simulink model "Question12_22104137"  (R2022a)
settings: Solver=ode3  StartTime=0.0  StopTime=0.5  FixedStep=T  RelTol=1e-3
InitFcn:
  | T=5e-6
  | fsw=1550
  | Ts=1/fsw
libraries: spsDiodeLib x18, spsIGBTDiodeLib x8, spsCurrentMeasurementLib x7, spsSeriesRLCBranchLib x7, simulink x6, spsVoltageMeasurementLib x4, spsMeanLib x3, spsMultiWindingTransformerLib x3, spsThreePhaseSourceLib x1, spspowerguiLib x1
settings Model: Creator=vinay  LastModifiedBy=vinay
settings DataIOCC: SaveFormat=StructureWithTime  ReturnWorkspaceOutputs=off
settings ModelReferenceCC: EnableRefExpFcnMdlSchedulingChecks=off
settings RTWCC: Description=Generic Real-Time Target

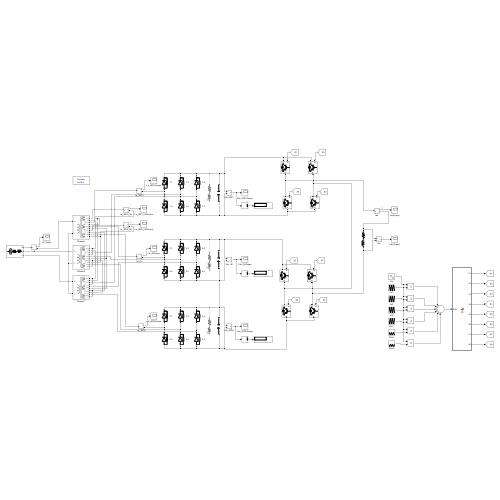
[thumbnail: Simulink's stored preview of the top-level diagram]
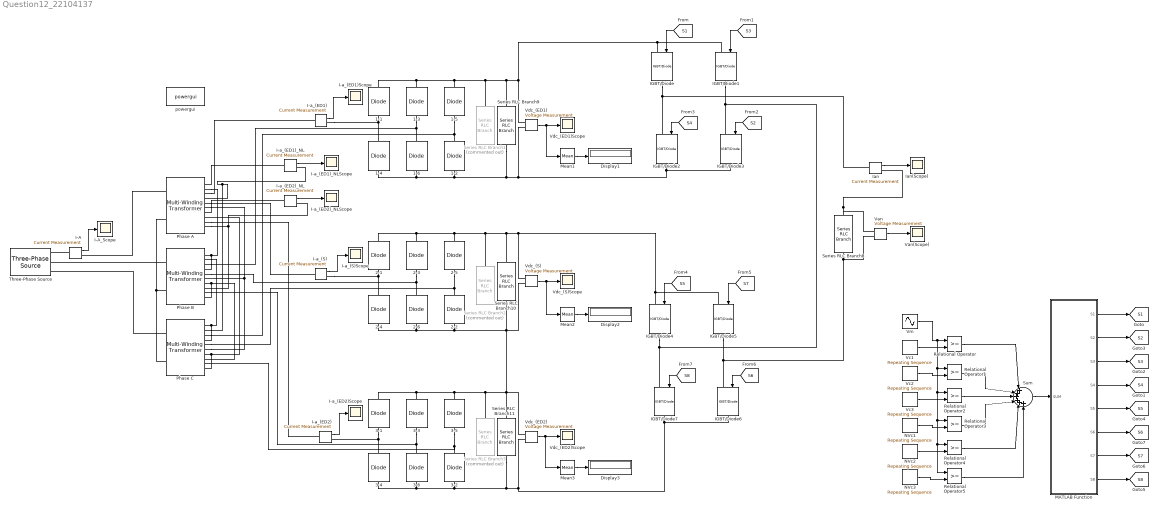
== system Question12_22104137 ==
  1-{1..6} (6 alike) : spsDiodeLib/Diode  Ron=0.001  Lon=0  Vf=0.8  IC=0  UseSnubber=0  Rs=500  Cs=250e-9  Measurements=off
  2-{1..6} (6 alike) : spsDiodeLib/Diode  Ron=0.001  Lon=0  Vf=0.8  IC=0  UseSnubber=0  Rs=500  Cs=250e-9  Measurements=off
  3-{1..6} (6 alike) : spsDiodeLib/Diode  Ron=0.001  Lon=0  Vf=0.8  IC=0  UseSnubber=0  Rs=500  Cs=250e-9  Measurements=off
  Display1 : Display
  Display2 : Display
  Display3 : Display
  I-A : spsCurrentMeasurementLib/Current Measurement  PhasorSimulation=off  OutputType=Complex  PSBequivalent=0
  I-A_Scope : Scope
  I-a_(ED1) : spsCurrentMeasurementLib/Current Measurement  PhasorSimulation=off  OutputType=Complex  PSBequivalent=0
  I-a_(ED1)Scope : Scope
  I-a_(ED1)_NL : spsCurrentMeasurementLib/Current Measurement  PhasorSimulation=off  OutputType=Complex  PSBequivalent=0
  I-a_(ED1)_NLScope : Scope
  I-a_(ED2) : spsCurrentMeasurementLib/Current Measurement  PhasorSimulation=off  OutputType=Complex  PSBequivalent=0
  I-a_(ED2)Scope : Scope
  I-a_(ED2)_NL : spsCurrentMeasurementLib/Current Measurement  PhasorSimulation=off  OutputType=Complex  PSBequivalent=0
  I-a_(ED2)_NLScope : Scope
  I-a_(S) : spsCurrentMeasurementLib/Current Measurement  PhasorSimulation=off  OutputType=Complex  PSBequivalent=0
  I-a_(S)Scope : Scope
  IGBT/Diode{,1..7} (8 alike) : spsIGBTDiodeLib/IGBT//Diode  Ron=1e-3  Rs=1e5  Cs=inf  Measurements=off
  Ian : spsCurrentMeasurementLib/Current Measurement  PhasorSimulation=off  OutputType=Complex  PSBequivalent=0
  Ian(Scope) : Scope
  MATLAB Function : MATLAB Function  TreatAsAtomicUnit=on
  Mean1 : spsMeanLib/Mean  Freq=50  Vinit=0  Ts=0
  Mean2 : spsMeanLib/Mean  Freq=50  Vinit=0  Ts=0
  Mean3 : spsMeanLib/Mean  Freq=50  Vinit=0  Ts=0
  NVc1 : simulink/Sources/Repeating Sequence  rep_seq_t=[0 1/2 1]*Ts  rep_seq_y=[0 -1 0]
  NVc2 : simulink/Sources/Repeating Sequence  rep_seq_t=[0 1/2 1]*Ts  rep_seq_y=[-2 -1 -2]
  NVc3 : simulink/Sources/Repeating Sequence  rep_seq_t=[0 1/2 1]*Ts  rep_seq_y=[-2 -3 -2]
  Phase A : spsMultiWindingTransformerLib/Multi-Winding Transformer  LeftWindings=1  RightWindings=5  TappedWindings=no taps  NumberOfTaps=2  SetSaturation=off  Hysteresis=off  DataFile='hysteresis.mat'  Measurements=None  UNITS=pu  NominalPower=[2.5e3 50]  NominalVoltages="[ 239.6  78.8  45.5  86  78.8  45.5 ]"  WindingResistances="[ 0  0  0  0  0  0 ]"  WindingInductances="[ 0.09  0.09  0.09  0.09  0.09  0.09 ]"  Rm=500  Lm=500  Saturation=[ 0,0 ; 0.0024,1.2 ; 1.0,1.52 ]  SpecifyInitialFlux=off  InitialFlux=0  BreakLoop=off  DiscreteSolver=Trapezoidal iterative  DataType=off  TransfoNumber=1
  Phase B : spsMultiWindingTransformerLib/Multi-Winding Transformer  LeftWindings=1  RightWindings=5  TappedWindings=no taps  NumberOfTaps=2  SetSaturation=off  Hysteresis=off  DataFile='hysteresis.mat'  Measurements=None  UNITS=pu  NominalPower=[2.5e3 50]  NominalVoltages="[ 239.6  78.8  45.5  86  78.8  45.5 ]"  WindingResistances="[ 0  0  0  0  0  0 ]"  WindingInductances="[ 0.09  0.09  0.09  0.09  0.09  0.09 ]"  Rm=500  Lm=500  Saturation=[ 0,0 ; 0.0024,1.2 ; 1.0,1.52 ]  SpecifyInitialFlux=off  InitialFlux=0  BreakLoop=off  DiscreteSolver=Trapezoidal iterative  DataType=off  TransfoNumber=1
  Phase C : spsMultiWindingTransformerLib/Multi-Winding Transformer  LeftWindings=1  RightWindings=5  TappedWindings=no taps  NumberOfTaps=2  SetSaturation=off  Hysteresis=off  DataFile='hysteresis.mat'  Measurements=None  UNITS=pu  NominalPower=[2.5e3 50]  NominalVoltages="[ 239.6  78.8  45.5  86  78.8  45.5 ]"  WindingResistances="[ 0  0  0  0  0  0 ]"  WindingInductances="[ 0.09  0.09  0.09  0.09  0.09  0.09 ]"  Rm=500  Lm=500  Saturation=[ 0,0 ; 0.0024,1.2 ; 1.0,1.52 ]  SpecifyInitialFlux=off  InitialFlux=0  BreakLoop=off  DiscreteSolver=Trapezoidal iterative  DataType=off  TransfoNumber=1
  Relational Operator{,1..5} (6 alike) : RelationalOperator  OutDataTypeStr=boolean  RndMeth=Simplest  InputSameDT=off
  Series RLC Branch1 : spsSeriesRLCBranchLib/Series RLC Branch  Commented=on  LConnTagsString=__new0  RConnTagsString=__new0  BranchType=RL  Resistance=50  Inductance=100e-3  SetiL0=off  InitialCurrent=0  Capacitance=1e-6  Setx0=off  InitialVoltage=0  Measurements=None
  Series RLC Branch10 : spsSeriesRLCBranchLib/Series RLC Branch  LConnTagsString=__new0  RConnTagsString=__new0  BranchType=C  Resistance=1  Inductance=1e-3  SetiL0=off  InitialCurrent=0  Capacitance=4700e-6  Setx0=off  InitialVoltage=0  Measurements=None
  Series RLC Branch11 : spsSeriesRLCBranchLib/Series RLC Branch  LConnTagsString=__new0  RConnTagsString=__new0  BranchType=C  Resistance=1  Inductance=1e-3  SetiL0=off  InitialCurrent=0  Capacitance=4700e-6  Setx0=off  InitialVoltage=0  Measurements=None
  Series RLC Branch2 : spsSeriesRLCBranchLib/Series RLC Branch  Commented=on  LConnTagsString=__new0  RConnTagsString=__new0  BranchType=RL  Resistance=50  Inductance=100e-3  SetiL0=off  InitialCurrent=0  Capacitance=1e-6  Setx0=off  InitialVoltage=0  Measurements=None
  Series RLC Branch3 : spsSeriesRLCBranchLib/Series RLC Branch  Commented=on  LConnTagsString=__new0  RConnTagsString=__new0  BranchType=RL  Resistance=50  Inductance=100e-3  SetiL0=off  InitialCurrent=0  Capacitance=1e-6  Setx0=off  InitialVoltage=0  Measurements=None
  Series RLC Branch8 : spsSeriesRLCBranchLib/Series RLC Branch  LConnTagsString=__new0  RConnTagsString=__new0  BranchType=RL  Resistance=50  Inductance=10e-3  SetiL0=off  InitialCurrent=0  Capacitance=1e-6  Setx0=off  InitialVoltage=0  Measurements=None
  Series RLC Branch9 : spsSeriesRLCBranchLib/Series RLC Branch  LConnTagsString=__new0  RConnTagsString=__new0  BranchType=C  Resistance=1  Inductance=1e-3  SetiL0=off  InitialCurrent=0  Capacitance=4700e-6  Setx0=off  InitialVoltage=0  Measurements=None
  Sum : Sum  Inputs=|++++++
  Three-Phase Source : spsThreePhaseSourceLib/Three-Phase Source  InternalConnection=Y  VoltagePhases=on  Voltage=415  PhaseAngle=0  Voltage_phases=[415 415 415]/sqrt(3)  PhaseAngles_phases=[0 120 240]  Frequency=50  NonIdealSource=on  SpecifyImpedance=off  Resistance=0.001  Inductance=5e-6  ShortCircuitLevel=100e6  BaseVoltage=415  XRratio=7  BusType=swing  Pref=10e3  Qref=0  Prefabc=[10e3, 10e3, 10e3]  Qrefabc=[0, 0, 0]  Qmin=-inf  Qmax=inf
  Van : spsVoltageMeasurementLib/Voltage Measurement  PhasorSimulation=off  OutputType=Complex  PSBequivalent=0
  Van(Scope) : Scope
  Vc1 : simulink/Sources/Repeating Sequence  rep_seq_t=[0 1/2 1]*Ts  rep_seq_y=[0 1 0]
  Vc2 : simulink/Sources/Repeating Sequence  rep_seq_t=[0 1/2 1]*Ts  rep_seq_y=[2 1 2]
  Vc3 : simulink/Sources/Repeating Sequence  rep_seq_t=[0 1/2 1]*Ts  rep_seq_y=[2 3 2]
  Vdc_(ED1) : spsVoltageMeasurementLib/Voltage Measurement  PhasorSimulation=off  OutputType=Complex  PSBequivalent=0
  Vdc_(ED1)Scope : Scope
  Vdc_(ED2) : spsVoltageMeasurementLib/Voltage Measurement  PhasorSimulation=off  OutputType=Complex  PSBequivalent=0
  Vdc_(ED2)Scope : Scope
  Vdc_(S) : spsVoltageMeasurementLib/Voltage Measurement  PhasorSimulation=off  OutputType=Complex  PSBequivalent=0
  Vdc_(S)Scope : Scope
  Vm : Sin  Amplitude=3  Frequency=2*pi*50  SampleTime=0
  powergui : spspowerguiLib/powergui  Priority=1  SimulationMode=Discrete  SampleTime=T  frequency=60  Iterations=50  frequencyindice=0  Pbase=100e6  ErrMax=1e-4  UnitsV=kV  UnitsW=MW  buscounter=0  FunctionMessages=off  echomessages=off  EnableUseOfTLC=off  CurrentSourceSwitches=off  DisableSnubberDevices=off  DisableRonSwitches=off  DisableVfSwitches=off  DisplayEquations=off  AutomaticDiscreteSolvers=off  SolverType=Tustin/Backward Euler (TBE)  Interpol=off  ExternalGateDelay=off  methode=off  Ts=100  x0status=blocks  SPID=on  SwTol=0  HookPort=off  NonlinearTolerance=1e-4  nMaxIteration=100  ContinueOnMaxIteration=off  RestoreLinks=warning  ResistiveCurrentMeasurement=off  Frange=[0:2:500]  Ylog=off  Xlog=on  ShowGrid=off  save=off  variable=ZData  structure=0  ZoomFFT=off  StartTime=0.0  cycles=1  DisplayStyle=1  fundamental=60  FreqAxis=off  MaxFrequency=1000  frequencyindicesteady=1  RmsSteady=1  display=off
  tag scope: S1=global, S2=global, S3=global, S4=global, S5=global, S6=global, S7=global, S8=global
  wires:
  Vdc_(ED1)/1 -> Vdc_(ED1)Scope/1, Mean1/1
  Mean1/1 -> Display1/1
  Vdc_(S)/1 -> Vdc_(S)Scope/1, Mean2/1
  Mean2/1 -> Display2/1
  Vdc_(ED2)/1 -> Vdc_(ED2)Scope/1, Mean3/1
  Mean3/1 -> Display3/1
  I-a_(ED1)/1 -> I-a_(ED1)Scope/1
  I-a_(S)/1 -> I-a_(S)Scope/1
  I-a_(ED2)/1 -> I-a_(ED2)Scope/1
  Van/1 -> Van(Scope)/1
  [S6] -> IGBT/Diode6/1
  [S7] -> IGBT/Diode5/1
  [S5] -> IGBT/Diode4/1
  Ian/1 -> Ian(Scope)/1
  [S2] -> IGBT/Diode3/1
  [S4] -> IGBT/Diode2/1
  [S8] -> IGBT/Diode7/1
  [S3] -> IGBT/Diode1/1
  [S1] -> IGBT/Diode/1
  I-A/1 -> I-A_Scope/1
  Vm/1 -> Relational Operator5/1, Relational Operator4/1, Relational Operator3/1, Relational Operator2/1, Relational Operator1/1, Relational Operator/1
  NVc3/1 -> Relational Operator5/2
  NVc2/1 -> Relational Operator4/2
  NVc1/1 -> Relational Operator3/2
  Vc3/1 -> Relational Operator2/2
  Vc2/1 -> Relational Operator1/2
  Vc1/1 -> Relational Operator/2
  Relational Operator/1 -> Sum/1
  Relational Operator1/1 -> Sum/2
  Relational Operator2/1 -> Sum/3
  Relational Operator3/1 -> Sum/4
  Relational Operator4/1 -> Sum/5
  Relational Operator5/1 -> Sum/6
  Sum/1 -> MATLAB Function/1(SUM)
  MATLAB Function/6(S6) -> [S6]
  MATLAB Function/1(S1) -> [S1]
  MATLAB Function/2(S2) -> [S2]
  MATLAB Function/3(S3) -> [S3]
  MATLAB Function/4(S4) -> [S4]
  MATLAB Function/5(S5) -> [S5]
  MATLAB Function/7(S7) -> [S7]
  MATLAB Function/8(S8) -> [S8]
  I-a_(ED1)_NL/1 -> I-a_(ED1)_NLScope/1
  I-a_(ED2)_NL/1 -> I-a_(ED2)_NLScope/1
  connections:
  1-1/LConn1 -- 1-4/RConn1 -- I-a_(ED1)/RConn1
  1-5/LConn1 -- Phase C/RConn3 -- 1-2/RConn1
  1-3/LConn1 -- Phase B/RConn3 -- 1-6/RConn1
  3-1/LConn1 -- 3-4/RConn1 -- I-a_(ED2)/RConn1
  3-5/LConn1 -- Phase C/RConn9 -- 3-2/RConn1
  3-3/LConn1 -- Phase B/RConn9 -- 3-6/RConn1
  2-1/LConn1 -- 2-4/RConn1 -- I-a_(S)/RConn1
  2-3/LConn1 -- Phase B/RConn5 -- 2-6/RConn1
  2-5/LConn1 -- Phase C/RConn5 -- 2-2/RConn1
  Vdc_(ED2)/LConn1 -- Series RLC Branch11/LConn1 -- Series RLC Branch10/RConn1 -- Vdc_(S)/LConn2 -- 2-4/LConn1 -- 2-6/LConn1 -- 2-2/LConn1 -- Series RLC Branch3/LConn1 -- 3-3/RConn1 -- 3-1/RConn1 -- 3-5/RConn1
  Ian/LConn1 -- IGBT/Diode2/LConn1 -- IGBT/Diode/RConn1
  Series RLC Branch8/RConn1 -- IGBT/Diode6/LConn1 -- IGBT/Diode5/RConn1 -- Van/LConn2
  IGBT/Diode7/LConn1 -- IGBT/Diode4/RConn1 -- IGBT/Diode3/LConn1 -- IGBT/Diode1/RConn1
  Phase B/LConn2 -- Phase A/LConn2 -- Phase C/LConn2
  Phase C/LConn1 -- Three-Phase Source/RConn3
  Phase A/LConn1 -- I-A/RConn1
  Phase B/LConn1 -- Three-Phase Source/RConn2
  I-A/LConn1 -- Three-Phase Source/RConn1
  Phase A/RConn1 -- I-a_(ED1)_NL/LConn1
  Phase B/RConn1 -- Phase A/RConn2 -- Phase B/RConn4
  Phase C/RConn1 -- Phase B/RConn2 -- Phase C/RConn4
  Phase A/RConn10 -- I-a_(ED2)_NL/RConn1 -- Phase B/RConn8
  Phase B/RConn7 -- Phase B/RConn10 -- Phase C/RConn8
  Phase C/RConn7 -- Phase C/RConn10 -- Phase A/RConn8
  Phase A/RConn6 -- Phase C/RConn6 -- Phase B/RConn6
  Phase A/RConn3 -- I-a_(ED1)/LConn1
  Phase A/RConn5 -- I-a_(S)/LConn1
  Phase A/RConn9 -- I-a_(ED2)/LConn1
  IGBT/Diode6/RConn1 -- Series RLC Branch11/RConn1 -- 3-2/LConn1 -- 3-4/LConn1 -- 3-6/LConn1 -- Vdc_(ED2)/LConn2 -- IGBT/Diode7/RConn1
  2-5/RConn1 -- Series RLC Branch2/LConn1 -- Vdc_(S)/LConn1 -- IGBT/Diode5/LConn1 -- IGBT/Diode4/LConn1 -- Series RLC Branch10/LConn1 -- 2-1/RConn1 -- 2-3/RConn1
  Series RLC Branch9/RConn1 -- Vdc_(ED1)/LConn2 -- IGBT/Diode3/RConn1 -- IGBT/Diode2/RConn1 -- 1-2/LConn1 -- 1-4/LConn1 -- 1-6/LConn1
  1-1/RConn1 -- Series RLC Branch9/LConn1 -- Vdc_(ED1)/LConn1 -- IGBT/Diode1/LConn1 -- IGBT/Diode/LConn1 -- Series RLC Branch1/LConn1 -- 1-5/RConn1 -- 1-3/RConn1
  Van/LConn1 -- Series RLC Branch8/LConn1 -- Ian/RConn1
  I-a_(ED1)_NL/RConn1 -- Phase C/RConn2 -- Phase A/RConn4
  I-a_(ED2)_NL/LConn1 -- Phase A/RConn7

== matlab function Question12_22104137/MATLAB Function ==
  data: SUM input; S1 output; S2 output; S3 output; S4 output; S5 output; S6 output; S7 output; S8 output
function [S1, S2, S3, S4, S5, S6, S7, S8] = fcn(SUM)  

S1=0;
S2=0;
S3=0;
S4=0;
S5=0;
S6=0;
S7=0;
S8=0;

if (SUM==6) %Van=+3E 
S1=1;
S2=1;
S3=0;
S4=0;
S5=1;
S6=1;
S7=0;
S8=0;

elseif (SUM==5) %Van=+2E  
S1=1;
S2=0;
S3=1;
S4=0;
S5=1;
S6=1;
S7=0;
S8=0;

elseif (SUM==4)  %Van=+E
S1=1;
S2=1;
S3=0;
S4=0;
S5=1;
S6=0;
S7=1;
S8=0;
    
elseif (SUM==3) %Van=0
S1=1;
S2=0;
S3=1;
S4=0;
S5=1;
S6=0;
S7=1;
S8=0;

elseif (SUM==2)  %Van=-E  
S1=0;
S2=0;
S3=1;
S4=1;
S5=1;
S6=0;
S7=1;
S8=0;
    
elseif (SUM==1) %Van=-2E  
S1=1;
S2=0;
S3=1;
S4=0;
S5=0;
S6=0;
S7=1;
S8=1;
    
elseif (SUM==0) %Van=-3E  
S1=0;
S2=0;
S3=1;
S4=1;
S5=0;
S6=0;
S7=1;
S8=1;

end
end
